simulink model "Eigenbewegung"  (R2021b)
settings: Solver=ode4  StartTime=0.0  StopTime=20  FixedStep=0.02  RelTol=1e-3
undefined symbols (not defined in the file): BFZ, ENV
settings Model: Creator=jonih  LastModifiedBy=jonih

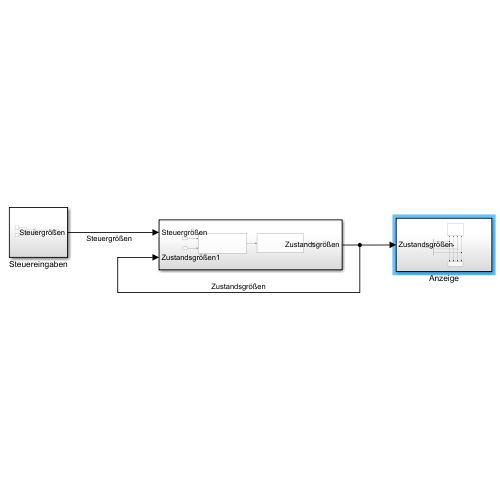
[thumbnail: Simulink's stored preview of the top-level diagram]
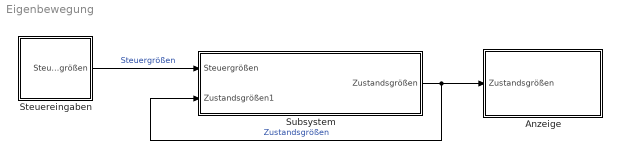
== system Eigenbewegung ==
  Anzeige : Subsystem
  Steuereingaben : Subsystem
  Subsystem : Subsystem
  wires:
  Steuereingaben/1(Steuergrößen) -> Subsystem/1(Steuergrößen)  "Steuergrößen"
  Subsystem/1(Zustandsgrößen) -> Anzeige/1(Zustandsgrößen), Subsystem/2(Zustandsgrößen1)  "Zustandsgrößen"

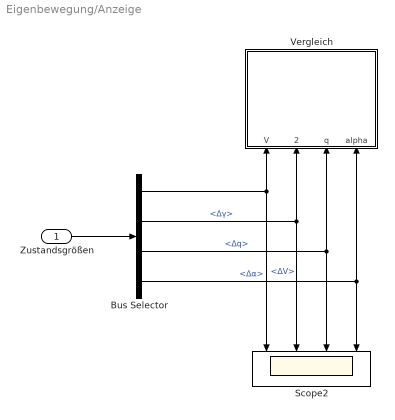
== system Eigenbewegung/Anzeige ==
  Zustandsgrößen : Inport
  Bus Selector : BusSelector  OutputSignals=ΔV,Δγ,Δq,Δα
  Scope2 : Scope  NumInputPorts=4
  Vergleich : Subsystem
  wires:
  Zustandsgrößen/1 -> Bus Selector/1
  Bus Selector/1 -> Vergleich/1(V), Scope2/1  "<ΔV>"
  Bus Selector/2 -> Vergleich/2(gamma), Scope2/2  "<Δγ>"
  Bus Selector/3 -> Vergleich/3(q), Scope2/3  "<Δq>"
  Bus Selector/4 -> Vergleich/4(alpha), Scope2/4  "<Δα>"

== system Eigenbewegung/Steuereingaben ==
  Bus Creator : BusCreator  Inputs=2
  Δδ : Constant  Value=0
  Δη : Constant  Value=0
  Steuergrößen : Outport
  wires:
  Δη/1 -> Bus Creator/1  "Δη"
  Δδ/1 -> Bus Creator/2  "Δδ"
  Bus Creator/1 -> Steuergrößen/1  "Steuergrößen"

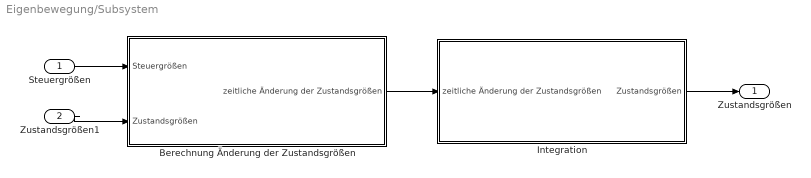
== system Eigenbewegung/Subsystem ==
  Steuergrößen : Inport
  Zustandsgrößen1 : Inport  Port=2
  Berechnung Änderung der Zustandsgrößen : Subsystem
  Integration : Subsystem
  Zustandsgrößen : Outport
  wires:
  Berechnung Änderung der Zustandsgrößen/1(zeitliche Änderung der Zustandsgrößen) -> Integration/1(zeitliche Änderung der Zustandsgrößen)
  Zustandsgrößen1/1 -> Berechnung Änderung der Zustandsgrößen/2(Zustandsgrößen)
  Integration/1(Zustandsgrößen) -> Zustandsgrößen/1
  Steuergrößen/1 -> Berechnung Änderung der Zustandsgrößen/1(Steuergrößen)

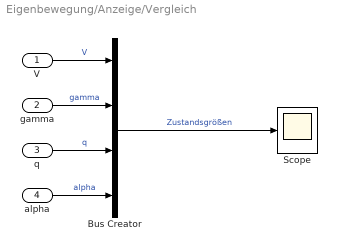
== system Eigenbewegung/Anzeige/Vergleich ==
  V : Inport
  gamma : Inport  Port=2
  q : Inport  Port=3
  alpha : Inport  Port=4
  Bus Creator : BusCreator  Inputs=4
  Scope : Scope
  wires:
  alpha/1 -> Bus Creator/4  "alpha"
  q/1 -> Bus Creator/3  "q"
  gamma/1 -> Bus Creator/2  "gamma"
  V/1 -> Bus Creator/1  "V"
  Bus Creator/1 -> Scope/1  "Zustandsgrößen"

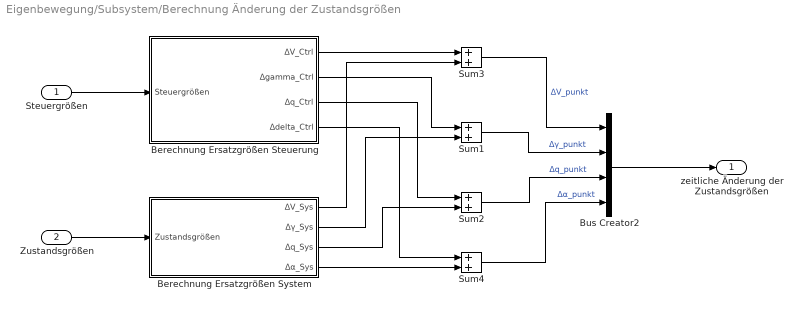
== system Eigenbewegung/Subsystem/Berechnung Änderung der Zustandsgrößen ==
  Steuergrößen : Inport
  Zustandsgrößen : Inport  Port=2
  Berechnung Ersatzgrößen Steuerung : Subsystem
  Berechnung Ersatzgrößen System : Subsystem
  Bus Creator2 : BusCreator  Inputs=4
  Sum1 : Sum
  Sum2 : Sum
  Sum3 : Sum
  Sum4 : Sum  Inputs=+|+
  zeitliche Änderung der Zustandsgrößen : Outport
  wires:
  Berechnung Ersatzgrößen Steuerung/3(Δq_Ctrl) -> Sum2/1
  Sum4/1 -> Bus Creator2/4  "Δα_punkt"
  Sum1/1 -> Bus Creator2/2  "Δγ_punkt"
  Sum2/1 -> Bus Creator2/3  "Δq_punkt"
  Sum3/1 -> Bus Creator2/1  "ΔV_punkt"
  Zustandsgrößen/1 -> Berechnung Ersatzgrößen System/1(Zustandsgrößen)
  Berechnung Ersatzgrößen System/4(Δα_Sys) -> Sum4/2
  Bus Creator2/1 -> zeitliche Änderung der Zustandsgrößen/1
  Berechnung Ersatzgrößen Steuerung/1(ΔV_Ctrl) -> Sum3/1
  Berechnung Ersatzgrößen Steuerung/4(Δdelta_Ctrl) -> Sum4/1
  Berechnung Ersatzgrößen System/1(ΔV_Sys) -> Sum3/2
  Berechnung Ersatzgrößen Steuerung/2(Δgamma_Ctrl) -> Sum1/1
  Steuergrößen/1 -> Berechnung Ersatzgrößen Steuerung/1(Steuergrößen)
  Berechnung Ersatzgrößen System/2(Δγ_Sys) -> Sum1/2
  Berechnung Ersatzgrößen System/3(Δq_Sys) -> Sum2/2

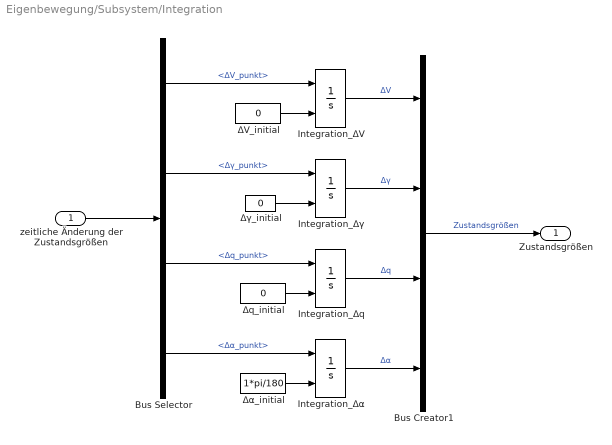
== system Eigenbewegung/Subsystem/Integration ==
  zeitliche Änderung der Zustandsgrößen : Inport
  Bus Creator1 : BusCreator  Inputs=4
  Bus Selector : BusSelector  OutputSignals=ΔV_punkt,Δγ_punkt,Δq_punkt,Δα_punkt
  Integration_ΔV : Integrator  InitialConditionSource=external
  Integration_Δq : Integrator  InitialConditionSource=external
  Integration_Δα : Integrator  InitialConditionSource=external
  Integration_Δγ : Integrator  InitialConditionSource=external
  ΔV_initial : Constant  Value=0
  Δq_initial : Constant  Value=0
  Δα_initial : Constant  Value=1*pi/180
  Δγ_initial : Constant  Value=0
  Zustandsgrößen : Outport
  wires:
  zeitliche Änderung der Zustandsgrößen/1 -> Bus Selector/1
  Bus Selector/3 -> Integration_Δq/1  "<Δq_punkt>"
  Bus Selector/4 -> Integration_Δα/1  "<Δα_punkt>"
  Integration_Δγ/1 -> Bus Creator1/2  "Δγ"
  Integration_ΔV/1 -> Bus Creator1/1  "ΔV"
  Bus Selector/1 -> Integration_ΔV/1  "<ΔV_punkt>"
  Integration_Δq/1 -> Bus Creator1/3  "Δq"
  Bus Selector/2 -> Integration_Δγ/1  "<Δγ_punkt>"
  Integration_Δα/1 -> Bus Creator1/4  "Δα"
  Δγ_initial/1 -> Integration_Δγ/2
  Δα_initial/1 -> Integration_Δα/2
  Δq_initial/1 -> Integration_Δq/2
  ΔV_initial/1 -> Integration_ΔV/2
  Bus Creator1/1 -> Zustandsgrößen/1  "Zustandsgrößen"

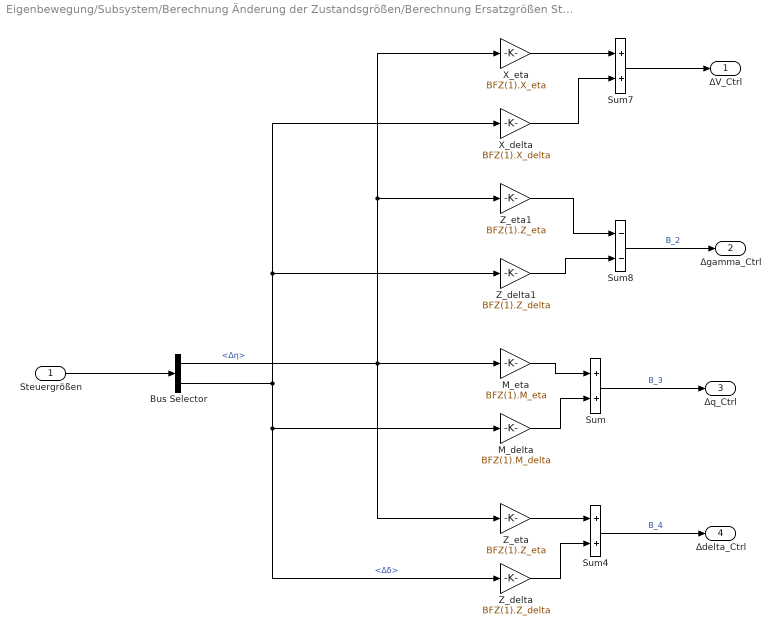
== system Eigenbewegung/Subsystem/Berechnung Änderung der Zustandsgrößen/Berechnung Ersatzgrößen Steuerung ==
  Steuergrößen : Inport
  Bus Selector : BusSelector  OutputSignals=Δη,Δδ
  M_delta : Gain  Gain=BFZ(1).M_delta
  M_eta : Gain  Gain=BFZ(1).M_eta
  Sum : Sum
  Sum4 : Sum
  Sum7 : Sum
  Sum8 : Sum  Inputs=--
  X_delta : Gain  Gain=BFZ(1).X_delta
  X_eta : Gain  Gain=BFZ(1).X_eta
  Z_delta : Gain  Gain=BFZ(1).Z_delta
  Z_delta1 : Gain  Gain=BFZ(1).Z_delta
  Z_eta : Gain  Gain=BFZ(1).Z_eta
  Z_eta1 : Gain  Gain=BFZ(1).Z_eta
  ΔV_Ctrl : Outport
  Δgamma_Ctrl : Outport  Port=2
  Δq_Ctrl : Outport  Port=3
  Δdelta_Ctrl : Outport  Port=4
  wires:
  Z_eta/1 -> Sum4/1
  M_eta/1 -> Sum/1
  Z_eta1/1 -> Sum8/1
  Z_delta/1 -> Sum4/2
  Bus Selector/2 -> M_delta/1, Z_delta/1, Z_delta1/1, X_delta/1  "<Δδ>"
  M_delta/1 -> Sum/2
  X_delta/1 -> Sum7/2
  Sum4/1 -> Δdelta_Ctrl/1  "B_4"
  Z_delta1/1 -> Sum8/2
  X_eta/1 -> Sum7/1
  Sum7/1 -> ΔV_Ctrl/1
  Sum8/1 -> Δgamma_Ctrl/1  "B_2"
  Sum/1 -> Δq_Ctrl/1  "B_3"
  Steuergrößen/1 -> Bus Selector/1
  Bus Selector/1 -> X_eta/1, Z_eta1/1, Z_eta/1, M_eta/1  "<Δη>"

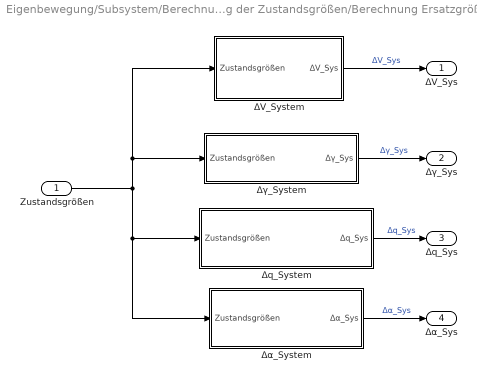
== system Eigenbewegung/Subsystem/Berechnung Änderung der Zustandsgrößen/Berechnung Ersatzgrößen System ==
  Zustandsgrößen : Inport
  ΔV_System : Subsystem
  Δq_System : Subsystem
  Δα_System : Subsystem
  Δγ_System : Subsystem
  ΔV_Sys : Outport
  Δγ_Sys : Outport  Port=2
  Δq_Sys : Outport  Port=3
  Δα_Sys : Outport  Port=4
  wires:
  Δγ_System/1(Δγ_Sys) -> Δγ_Sys/1  "Δγ_Sys"
  Zustandsgrößen/1 -> Δγ_System/1(Zustandsgrößen), ΔV_System/1(Zustandsgrößen), Δq_System/1(Zustandsgrößen), Δα_System/1(Zustandsgrößen)
  Δα_System/1(Δα_Sys) -> Δα_Sys/1  "Δα_Sys"
  Δq_System/1(Δq_Sys) -> Δq_Sys/1  "Δq_Sys"
  ΔV_System/1(ΔV_Sys) -> ΔV_Sys/1  "ΔV_Sys"

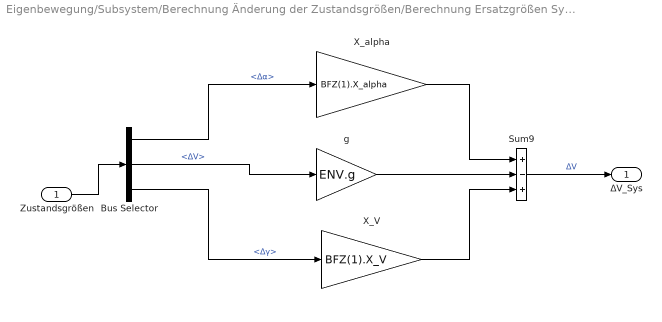
== system Eigenbewegung/Subsystem/Berechnung Änderung der Zustandsgrößen/Berechnung Ersatzgrößen System/ΔV_System ==
  Zustandsgrößen : Inport
  Bus Selector : BusSelector  OutputSignals=Δα,ΔV,Δγ
  Sum9 : Sum  Inputs=+-+
  X_V : Gain  Gain=BFZ(1).X_V
  X_alpha : Gain  Gain=BFZ(1).X_alpha
  g : Gain  Gain=ENV.g
  ΔV_Sys : Outport
  wires:
  Bus Selector/3 -> X_V/1  "<Δγ>"
  Bus Selector/1 -> X_alpha/1  "<Δα>"
  Sum9/1 -> ΔV_Sys/1  "ΔV"
  Bus Selector/2 -> g/1  "<ΔV>"
  g/1 -> Sum9/2
  Zustandsgrößen/1 -> Bus Selector/1
  X_V/1 -> Sum9/3
  X_alpha/1 -> Sum9/1

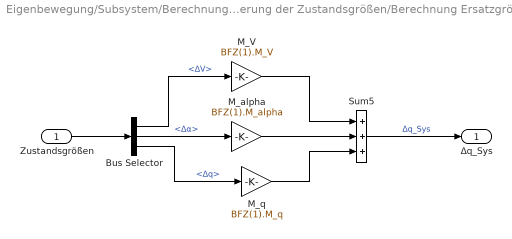
== system Eigenbewegung/Subsystem/Berechnung Änderung der Zustandsgrößen/Berechnung Ersatzgrößen System/Δq_System ==
  Zustandsgrößen : Inport
  Bus Selector : BusSelector  OutputSignals=ΔV,Δα,Δq
  M_V : Gain  Gain=BFZ(1).M_V
  M_alpha : Gain  Gain=BFZ(1).M_alpha
  M_q : Gain  Gain=BFZ(1).M_q
  Sum5 : Sum  Inputs=+++
  Δq_Sys : Outport
  wires:
  Bus Selector/2 -> M_alpha/1  "<Δα>"
  Bus Selector/1 -> M_V/1  "<ΔV>"
  Sum5/1 -> Δq_Sys/1  "Δq_Sys"
  Bus Selector/3 -> M_q/1  "<Δq>"
  Zustandsgrößen/1 -> Bus Selector/1
  M_alpha/1 -> Sum5/2
  M_V/1 -> Sum5/1
  M_q/1 -> Sum5/3

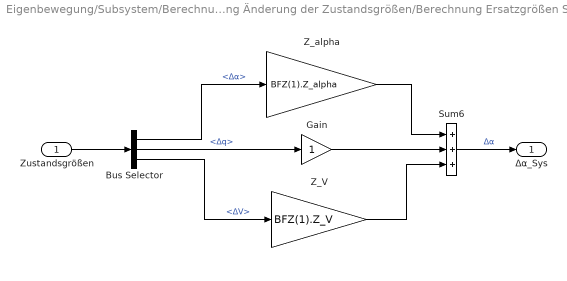
== system Eigenbewegung/Subsystem/Berechnung Änderung der Zustandsgrößen/Berechnung Ersatzgrößen System/Δα_System ==
  Zustandsgrößen : Inport
  Bus Selector : BusSelector  OutputSignals=Δα,Δq,ΔV
  Gain : Gain
  Sum6 : Sum  Inputs=+++
  Z_V : Gain  Gain=BFZ(1).Z_V
  Z_alpha : Gain  Gain=BFZ(1).Z_alpha
  Δα_Sys : Outport
  wires:
  Bus Selector/1 -> Z_alpha/1  "<Δα>"
  Bus Selector/2 -> Gain/1  "<Δq>"
  Bus Selector/3 -> Z_V/1  "<ΔV>"
  Sum6/1 -> Δα_Sys/1  "Δα"
  Z_alpha/1 -> Sum6/1
  Gain/1 -> Sum6/2
  Z_V/1 -> Sum6/3
  Zustandsgrößen/1 -> Bus Selector/1

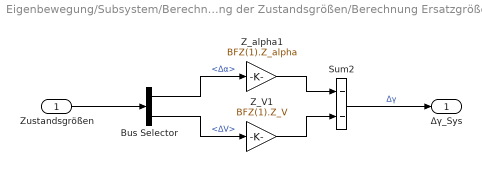
== system Eigenbewegung/Subsystem/Berechnung Änderung der Zustandsgrößen/Berechnung Ersatzgrößen System/Δγ_System ==
  Zustandsgrößen : Inport
  Bus Selector : BusSelector  OutputSignals=Δα,ΔV
  Sum2 : Sum  Inputs=--
  Z_V1 : Gain  Gain=BFZ(1).Z_V
  Z_alpha1 : Gain  Gain=BFZ(1).Z_alpha
  Δγ_Sys : Outport
  wires:
  Bus Selector/2 -> Z_V1/1  "<ΔV>"
  Bus Selector/1 -> Z_alpha1/1  "<Δα>"
  Sum2/1 -> Δγ_Sys/1  "Δγ"
  Zustandsgrößen/1 -> Bus Selector/1
  Z_alpha1/1 -> Sum2/1
  Z_V1/1 -> Sum2/2
